simulink model "sg_2d_fir"  (Simulink 7.6)
settings: Solver=ode45  StartTime=0.0  StopTime=1600.0  RelTol=1e-3
undefined symbols (not defined in the file): gcbh, xlBlockLoadCallback, xlGetNormalizedPeriod, xlipgetpartsetting
libraries: xbsIndex_r4 x311, dspsrcs4 x6
(part 4 of 4)

== system sg_2d_fir/sg_2d_fir/5x5_Filters/Green_Filter/5x5_Filter/2D_FIR/n-tap FIR Compiler Filter4 ==
  Din : Inport
  coef : Inport  Port=2
  load : Inport  Port=3
  "FIR Compiler 5.0 " : xbsIndex_r4/FIR Compiler 5.0   coefficientvector=zeros(1,5)  coefficient_sets=1  filter_type=Single_Rate  rate_change_type=Integer  interpolation_rate=1  decimation_rate=1  zero_pack_factor=1  number_channels=1  ratespecification=Maximum_Possible  sampleperiod=1  hardwareoversamplingrate=1  filter_architecture=Systolic_Multiply_Accumulate  coefficient_reload=on  coefficient_structure=Non_Symmetric  coefficient_sign=Signed  quantization=Quantize_Only  coefficient_width=coef_n_bits  bestprecision=off  coefficient_fractional_bits=coef_bin_pt  number_paths=1  output_rounding_mode=Full_Precision  output_width=26  allow_rounding_approximation=off  optimization_goal=Area  has_sclr=off  has_data_valid=off  has_nd=off  has_ce=off  usechan_in_adv=off  chan_in_adv=0  data_buffer_type=Automatic  coefficient_buffer_type=Automatic  input_buffer_type=Automatic  output_buffer_type=Automatic  preference_for_other_storage=Automatic  multi_column_support=Disabled  columnconfig='1'  inter_column_pipe_length=4  passband_min=0.0  passband_max=0.5  stopband_min=0.5  stopband_max=1.0  filter_selection=1  gui_behaviour=Sysgen  registered_output=true  data_sign=Signed  data_width=16  data_fractional_bits=0  wrapper_available=true  ip_wrap_arbitrary_binary_point=true  ip_name=FIR Compiler  ip_version=5.0  dsptool_ready=true  ipcore_usecache=true  ipcore_useipmodelcache=true  ipcore_xco_need_fpga_part=true  port_translation_map={ 'ce' => 'en', 'sclr' => 'rst' }  run_core_at_system_period=true  ipcore_fpga_part=xlipgetpartsetting(gcb, {'virtex4', 'xc4vsx35', '-10', 'ff668'})  structural_sim=false  block_type=fir_compiler_v5_0
      settings: block_version=11.2
  Register : xbsIndex_r4/Register  init=0  rst=off  en=on  dbl_ovrd=off  block_type=register
  Register2 : xbsIndex_r4/Register  init=0  rst=off  en=off  dbl_ovrd=off  block_type=register
      settings: block_version=9.1-beta
  Rising Edge Detector1 : Subsystem
  Terminator5 : Terminator
  Out : Outport
  wires:
  "FIR Compiler 5.0 "/2 -> Terminator5/1
  Rising Edge Detector1/1(Dout) -> "FIR Compiler 5.0 "/2
  Register2/1 -> "FIR Compiler 5.0 "/3
  load/1 -> Rising Edge Detector1/1(Din), Register2/1
  Register/1 -> Out/1
  coef/1 -> "FIR Compiler 5.0 "/4
  "FIR Compiler 5.0 "/1 -> Register/1
  "FIR Compiler 5.0 "/3 -> Register/2
  Din/1 -> "FIR Compiler 5.0 "/1

== system sg_2d_fir/sg_2d_fir/5x5_Filters/Green_Filter/5x5_Filter/2D_FIR/n-tap FIR Compiler Filter5 ==
  Din : Inport
  coef : Inport  Port=2
  load : Inport  Port=3
  "FIR Compiler 5.0 " : xbsIndex_r4/FIR Compiler 5.0   coefficientvector=zeros(1,5)  coefficient_sets=1  filter_type=Single_Rate  rate_change_type=Integer  interpolation_rate=1  decimation_rate=1  zero_pack_factor=1  number_channels=1  ratespecification=Maximum_Possible  sampleperiod=1  hardwareoversamplingrate=1  filter_architecture=Systolic_Multiply_Accumulate  coefficient_reload=on  coefficient_structure=Non_Symmetric  coefficient_sign=Signed  quantization=Quantize_Only  coefficient_width=coef_n_bits  bestprecision=off  coefficient_fractional_bits=coef_bin_pt  number_paths=1  output_rounding_mode=Full_Precision  output_width=26  allow_rounding_approximation=off  optimization_goal=Area  has_sclr=off  has_data_valid=off  has_nd=off  has_ce=off  usechan_in_adv=off  chan_in_adv=0  data_buffer_type=Automatic  coefficient_buffer_type=Automatic  input_buffer_type=Automatic  output_buffer_type=Automatic  preference_for_other_storage=Automatic  multi_column_support=Disabled  columnconfig='1'  inter_column_pipe_length=4  passband_min=0.0  passband_max=0.5  stopband_min=0.5  stopband_max=1.0  filter_selection=1  gui_behaviour=Sysgen  registered_output=true  data_sign=Signed  data_width=16  data_fractional_bits=0  wrapper_available=true  ip_wrap_arbitrary_binary_point=true  ip_name=FIR Compiler  ip_version=5.0  dsptool_ready=true  ipcore_usecache=true  ipcore_useipmodelcache=true  ipcore_xco_need_fpga_part=true  port_translation_map={ 'ce' => 'en', 'sclr' => 'rst' }  run_core_at_system_period=true  ipcore_fpga_part=xlipgetpartsetting(gcb, {'virtex4', 'xc4vsx35', '-10', 'ff668'})  structural_sim=false  block_type=fir_compiler_v5_0
      settings: block_version=11.2
  Register : xbsIndex_r4/Register  init=0  rst=off  en=on  dbl_ovrd=off  block_type=register
  Register2 : xbsIndex_r4/Register  init=0  rst=off  en=off  dbl_ovrd=off  block_type=register
      settings: block_version=9.1-beta
  Rising Edge Detector1 : Subsystem
  Terminator5 : Terminator
  Out : Outport
  wires:
  Din/1 -> "FIR Compiler 5.0 "/1
  "FIR Compiler 5.0 "/3 -> Register/2
  "FIR Compiler 5.0 "/1 -> Register/1
  coef/1 -> "FIR Compiler 5.0 "/4
  Register/1 -> Out/1
  load/1 -> Register2/1, Rising Edge Detector1/1(Din)
  Register2/1 -> "FIR Compiler 5.0 "/3
  Rising Edge Detector1/1(Dout) -> "FIR Compiler 5.0 "/2
  "FIR Compiler 5.0 "/2 -> Terminator5/1

== system sg_2d_fir/sg_2d_fir/5x5_Filters/Red_Filter/5x5_Filter/2D_FIR/ABS ==
  In1 : Inport
  Mux : xbsIndex_r4/Mux  inputs=2  en=off  latency=1  precision=Full  arith_type=Unsigned  n_bits=8  bin_pt=0  quantization=Truncate  overflow=Saturate  dbl_ovrd=off  block_type=mux
      settings: xl_area=[0, 0, 0, 0, 0, 0, 0]  block_version=VER_STRING_GOES_HERE
  Negate : xbsIndex_r4/Negate  precision=Full  arith_type=Unsigned  n_bits=8  bin_pt=2  quantization=Truncate  overflow=Wrap  en=off  latency=1  dbl_ovrd=off  block_type=negate
      settings: xl_area=[0, 0, 0, 0, 0, 0, 0]  block_version=VER_STRING_GOES_HERE
  Register1 : xbsIndex_r4/Register  init=0  rst=off  en=off  dbl_ovrd=off  block_type=register
      settings: xl_area=[0, 0, 0, 0, 0, 0, 0]  block_version=VER_STRING_GOES_HERE
  Register2 : xbsIndex_r4/Register  init=0  rst=off  en=off  dbl_ovrd=off  block_type=register
      settings: xl_area=[0, 0, 0, 0, 0, 0, 0]  block_version=VER_STRING_GOES_HERE
  Slice : xbsIndex_r4/Slice  nbits=1  boolean_output=off  mode=Upper Bit Location + Width  bit1=0  base1=MSB of Input  bit0=0  base0=LSB of Input  dbl_ovrd=off  block_type=slice
      settings: infoedit="Extracts a given range of bits from each input sample and presents it at the output.  The output type is ordinarily unsigned with binary point at zero, but can be Boolean when the slice is one bit wide.<P><P>Hardware notes: In hardware this block costs nothing."  block_version=VER_STRING_GOES_HERE
  Out1 : Outport
  wires:
  Register1/1 -> Mux/2
  Register2/1 -> Mux/1
  Mux/1 -> Out1/1
  In1/1 -> Register1/1, Slice/1, Negate/1
  Negate/1 -> Mux/3
  Slice/1 -> Register2/1

== system sg_2d_fir/sg_2d_fir/5x5_Filters/Red_Filter/5x5_Filter/2D_FIR/n-tap FIR Compiler Filter1 ==
  Din : Inport
  coef : Inport  Port=2
  load : Inport  Port=3
  "FIR Compiler 5.0 " : xbsIndex_r4/FIR Compiler 5.0   coefficientvector=zeros(1,5)  coefficient_sets=1  filter_type=Single_Rate  rate_change_type=Integer  interpolation_rate=1  decimation_rate=1  zero_pack_factor=1  number_channels=1  ratespecification=Maximum_Possible  sampleperiod=1  hardwareoversamplingrate=1  filter_architecture=Systolic_Multiply_Accumulate  coefficient_reload=on  coefficient_structure=Non_Symmetric  coefficient_sign=Signed  quantization=Quantize_Only  coefficient_width=coef_n_bits  bestprecision=off  coefficient_fractional_bits=coef_bin_pt  number_paths=1  output_rounding_mode=Full_Precision  output_width=26  allow_rounding_approximation=off  optimization_goal=Area  has_sclr=off  has_data_valid=off  has_nd=off  has_ce=off  usechan_in_adv=off  chan_in_adv=0  data_buffer_type=Automatic  coefficient_buffer_type=Automatic  input_buffer_type=Automatic  output_buffer_type=Automatic  preference_for_other_storage=Automatic  multi_column_support=Disabled  columnconfig='1'  inter_column_pipe_length=4  passband_min=0.0  passband_max=0.5  stopband_min=0.5  stopband_max=1.0  filter_selection=1  gui_behaviour=Sysgen  registered_output=true  data_sign=Signed  data_width=16  data_fractional_bits=0  wrapper_available=true  ip_wrap_arbitrary_binary_point=true  ip_name=FIR Compiler  ip_version=5.0  dsptool_ready=true  ipcore_usecache=true  ipcore_useipmodelcache=true  ipcore_xco_need_fpga_part=true  port_translation_map={ 'ce' => 'en', 'sclr' => 'rst' }  run_core_at_system_period=true  ipcore_fpga_part=xlipgetpartsetting(gcb, {'virtex4', 'xc4vsx35', '-10', 'ff668'})  structural_sim=false  block_type=fir_compiler_v5_0
      settings: block_version=11.2
  Register : xbsIndex_r4/Register  init=0  rst=off  en=on  dbl_ovrd=off  block_type=register
  Register2 : xbsIndex_r4/Register  init=0  rst=off  en=off  dbl_ovrd=off  block_type=register
      settings: block_version=9.1-beta
  Rising Edge Detector1 : Subsystem
  Terminator5 : Terminator
  Out : Outport
  wires:
  "FIR Compiler 5.0 "/2 -> Terminator5/1
  Rising Edge Detector1/1(Dout) -> "FIR Compiler 5.0 "/2
  Register2/1 -> "FIR Compiler 5.0 "/3
  load/1 -> Rising Edge Detector1/1(Din), Register2/1
  Register/1 -> Out/1
  coef/1 -> "FIR Compiler 5.0 "/4
  "FIR Compiler 5.0 "/1 -> Register/1
  "FIR Compiler 5.0 "/3 -> Register/2
  Din/1 -> "FIR Compiler 5.0 "/1

== system sg_2d_fir/sg_2d_fir/5x5_Filters/Red_Filter/5x5_Filter/2D_FIR/n-tap FIR Compiler Filter2 ==
  Din : Inport
  coef : Inport  Port=2
  load : Inport  Port=3
  "FIR Compiler 5.0 " : xbsIndex_r4/FIR Compiler 5.0   coefficientvector=zeros(1,5)  coefficient_sets=1  filter_type=Single_Rate  rate_change_type=Integer  interpolation_rate=1  decimation_rate=1  zero_pack_factor=1  number_channels=1  ratespecification=Maximum_Possible  sampleperiod=1  hardwareoversamplingrate=1  filter_architecture=Systolic_Multiply_Accumulate  coefficient_reload=on  coefficient_structure=Non_Symmetric  coefficient_sign=Signed  quantization=Quantize_Only  coefficient_width=coef_n_bits  bestprecision=off  coefficient_fractional_bits=coef_bin_pt  number_paths=1  output_rounding_mode=Full_Precision  output_width=26  allow_rounding_approximation=off  optimization_goal=Area  has_sclr=off  has_data_valid=off  has_nd=off  has_ce=off  usechan_in_adv=off  chan_in_adv=0  data_buffer_type=Automatic  coefficient_buffer_type=Automatic  input_buffer_type=Automatic  output_buffer_type=Automatic  preference_for_other_storage=Automatic  multi_column_support=Disabled  columnconfig='1'  inter_column_pipe_length=4  passband_min=0.0  passband_max=0.5  stopband_min=0.5  stopband_max=1.0  filter_selection=1  gui_behaviour=Sysgen  registered_output=true  data_sign=Signed  data_width=16  data_fractional_bits=0  wrapper_available=true  ip_wrap_arbitrary_binary_point=true  ip_name=FIR Compiler  ip_version=5.0  dsptool_ready=true  ipcore_usecache=true  ipcore_useipmodelcache=true  ipcore_xco_need_fpga_part=true  port_translation_map={ 'ce' => 'en', 'sclr' => 'rst' }  run_core_at_system_period=true  ipcore_fpga_part=xlipgetpartsetting(gcb, {'virtex4', 'xc4vsx35', '-10', 'ff668'})  structural_sim=false  block_type=fir_compiler_v5_0
      settings: block_version=11.2
  Register : xbsIndex_r4/Register  init=0  rst=off  en=on  dbl_ovrd=off  block_type=register
  Register2 : xbsIndex_r4/Register  init=0  rst=off  en=off  dbl_ovrd=off  block_type=register
      settings: block_version=9.1-beta
  Rising Edge Detector1 : Subsystem
  Terminator5 : Terminator
  Out : Outport
  wires:
  Din/1 -> "FIR Compiler 5.0 "/1
  "FIR Compiler 5.0 "/3 -> Register/2
  "FIR Compiler 5.0 "/1 -> Register/1
  coef/1 -> "FIR Compiler 5.0 "/4
  Register/1 -> Out/1
  load/1 -> Register2/1, Rising Edge Detector1/1(Din)
  Register2/1 -> "FIR Compiler 5.0 "/3
  Rising Edge Detector1/1(Dout) -> "FIR Compiler 5.0 "/2
  "FIR Compiler 5.0 "/2 -> Terminator5/1

== system sg_2d_fir/sg_2d_fir/5x5_Filters/Red_Filter/5x5_Filter/2D_FIR/n-tap FIR Compiler Filter3 ==
  Din : Inport
  coef : Inport  Port=2
  load : Inport  Port=3
  "FIR Compiler 5.0 " : xbsIndex_r4/FIR Compiler 5.0   coefficientvector=zeros(1,5)  coefficient_sets=1  filter_type=Single_Rate  rate_change_type=Integer  interpolation_rate=1  decimation_rate=1  zero_pack_factor=1  number_channels=1  ratespecification=Maximum_Possible  sampleperiod=1  hardwareoversamplingrate=1  filter_architecture=Systolic_Multiply_Accumulate  coefficient_reload=on  coefficient_structure=Non_Symmetric  coefficient_sign=Signed  quantization=Quantize_Only  coefficient_width=coef_n_bits  bestprecision=off  coefficient_fractional_bits=coef_bin_pt  number_paths=1  output_rounding_mode=Full_Precision  output_width=26  allow_rounding_approximation=off  optimization_goal=Area  has_sclr=off  has_data_valid=off  has_nd=off  has_ce=off  usechan_in_adv=off  chan_in_adv=0  data_buffer_type=Automatic  coefficient_buffer_type=Automatic  input_buffer_type=Automatic  output_buffer_type=Automatic  preference_for_other_storage=Automatic  multi_column_support=Disabled  columnconfig='1'  inter_column_pipe_length=4  passband_min=0.0  passband_max=0.5  stopband_min=0.5  stopband_max=1.0  filter_selection=1  gui_behaviour=Sysgen  registered_output=true  data_sign=Signed  data_width=16  data_fractional_bits=0  wrapper_available=true  ip_wrap_arbitrary_binary_point=true  ip_name=FIR Compiler  ip_version=5.0  dsptool_ready=true  ipcore_usecache=true  ipcore_useipmodelcache=true  ipcore_xco_need_fpga_part=true  port_translation_map={ 'ce' => 'en', 'sclr' => 'rst' }  run_core_at_system_period=true  ipcore_fpga_part=xlipgetpartsetting(gcb, {'virtex4', 'xc4vsx35', '-10', 'ff668'})  structural_sim=false  block_type=fir_compiler_v5_0
      settings: block_version=11.2
  Register : xbsIndex_r4/Register  init=0  rst=off  en=on  dbl_ovrd=off  block_type=register
  Register2 : xbsIndex_r4/Register  init=0  rst=off  en=off  dbl_ovrd=off  block_type=register
      settings: block_version=9.1-beta
  Rising Edge Detector1 : Subsystem
  Terminator5 : Terminator
  Out : Outport
  wires:
  "FIR Compiler 5.0 "/2 -> Terminator5/1
  Rising Edge Detector1/1(Dout) -> "FIR Compiler 5.0 "/2
  Register2/1 -> "FIR Compiler 5.0 "/3
  load/1 -> Rising Edge Detector1/1(Din), Register2/1
  Register/1 -> Out/1
  coef/1 -> "FIR Compiler 5.0 "/4
  "FIR Compiler 5.0 "/1 -> Register/1
  "FIR Compiler 5.0 "/3 -> Register/2
  Din/1 -> "FIR Compiler 5.0 "/1

== system sg_2d_fir/sg_2d_fir/5x5_Filters/Red_Filter/5x5_Filter/2D_FIR/n-tap FIR Compiler Filter4 ==
  Din : Inport
  coef : Inport  Port=2
  load : Inport  Port=3
  "FIR Compiler 5.0 " : xbsIndex_r4/FIR Compiler 5.0   coefficientvector=zeros(1,5)  coefficient_sets=1  filter_type=Single_Rate  rate_change_type=Integer  interpolation_rate=1  decimation_rate=1  zero_pack_factor=1  number_channels=1  ratespecification=Maximum_Possible  sampleperiod=1  hardwareoversamplingrate=1  filter_architecture=Systolic_Multiply_Accumulate  coefficient_reload=on  coefficient_structure=Non_Symmetric  coefficient_sign=Signed  quantization=Quantize_Only  coefficient_width=coef_n_bits  bestprecision=off  coefficient_fractional_bits=coef_bin_pt  number_paths=1  output_rounding_mode=Full_Precision  output_width=26  allow_rounding_approximation=off  optimization_goal=Area  has_sclr=off  has_data_valid=off  has_nd=off  has_ce=off  usechan_in_adv=off  chan_in_adv=0  data_buffer_type=Automatic  coefficient_buffer_type=Automatic  input_buffer_type=Automatic  output_buffer_type=Automatic  preference_for_other_storage=Automatic  multi_column_support=Disabled  columnconfig='1'  inter_column_pipe_length=4  passband_min=0.0  passband_max=0.5  stopband_min=0.5  stopband_max=1.0  filter_selection=1  gui_behaviour=Sysgen  registered_output=true  data_sign=Signed  data_width=16  data_fractional_bits=0  wrapper_available=true  ip_wrap_arbitrary_binary_point=true  ip_name=FIR Compiler  ip_version=5.0  dsptool_ready=true  ipcore_usecache=true  ipcore_useipmodelcache=true  ipcore_xco_need_fpga_part=true  port_translation_map={ 'ce' => 'en', 'sclr' => 'rst' }  run_core_at_system_period=true  ipcore_fpga_part=xlipgetpartsetting(gcb, {'virtex4', 'xc4vsx35', '-10', 'ff668'})  structural_sim=false  block_type=fir_compiler_v5_0
      settings: block_version=11.2
  Register : xbsIndex_r4/Register  init=0  rst=off  en=on  dbl_ovrd=off  block_type=register
  Register2 : xbsIndex_r4/Register  init=0  rst=off  en=off  dbl_ovrd=off  block_type=register
      settings: block_version=9.1-beta
  Rising Edge Detector1 : Subsystem
  Terminator5 : Terminator
  Out : Outport
  wires:
  Din/1 -> "FIR Compiler 5.0 "/1
  "FIR Compiler 5.0 "/3 -> Register/2
  "FIR Compiler 5.0 "/1 -> Register/1
  coef/1 -> "FIR Compiler 5.0 "/4
  Register/1 -> Out/1
  load/1 -> Register2/1, Rising Edge Detector1/1(Din)
  Register2/1 -> "FIR Compiler 5.0 "/3
  Rising Edge Detector1/1(Dout) -> "FIR Compiler 5.0 "/2
  "FIR Compiler 5.0 "/2 -> Terminator5/1

== system sg_2d_fir/sg_2d_fir/5x5_Filters/Red_Filter/5x5_Filter/2D_FIR/n-tap FIR Compiler Filter5 ==
  Din : Inport
  coef : Inport  Port=2
  load : Inport  Port=3
  "FIR Compiler 5.0 " : xbsIndex_r4/FIR Compiler 5.0   coefficientvector=zeros(1,5)  coefficient_sets=1  filter_type=Single_Rate  rate_change_type=Integer  interpolation_rate=1  decimation_rate=1  zero_pack_factor=1  number_channels=1  ratespecification=Maximum_Possible  sampleperiod=1  hardwareoversamplingrate=1  filter_architecture=Systolic_Multiply_Accumulate  coefficient_reload=on  coefficient_structure=Non_Symmetric  coefficient_sign=Signed  quantization=Quantize_Only  coefficient_width=coef_n_bits  bestprecision=off  coefficient_fractional_bits=coef_bin_pt  number_paths=1  output_rounding_mode=Full_Precision  output_width=26  allow_rounding_approximation=off  optimization_goal=Area  has_sclr=off  has_data_valid=off  has_nd=off  has_ce=off  usechan_in_adv=off  chan_in_adv=0  data_buffer_type=Automatic  coefficient_buffer_type=Automatic  input_buffer_type=Automatic  output_buffer_type=Automatic  preference_for_other_storage=Automatic  multi_column_support=Disabled  columnconfig='1'  inter_column_pipe_length=4  passband_min=0.0  passband_max=0.5  stopband_min=0.5  stopband_max=1.0  filter_selection=1  gui_behaviour=Sysgen  registered_output=true  data_sign=Signed  data_width=16  data_fractional_bits=0  wrapper_available=true  ip_wrap_arbitrary_binary_point=true  ip_name=FIR Compiler  ip_version=5.0  dsptool_ready=true  ipcore_usecache=true  ipcore_useipmodelcache=true  ipcore_xco_need_fpga_part=true  port_translation_map={ 'ce' => 'en', 'sclr' => 'rst' }  run_core_at_system_period=true  ipcore_fpga_part=xlipgetpartsetting(gcb, {'virtex4', 'xc4vsx35', '-10', 'ff668'})  structural_sim=false  block_type=fir_compiler_v5_0
      settings: block_version=11.2
  Register : xbsIndex_r4/Register  init=0  rst=off  en=on  dbl_ovrd=off  block_type=register
  Register2 : xbsIndex_r4/Register  init=0  rst=off  en=off  dbl_ovrd=off  block_type=register
      settings: block_version=9.1-beta
  Rising Edge Detector1 : Subsystem
  Terminator5 : Terminator
  Out : Outport
  wires:
  "FIR Compiler 5.0 "/2 -> Terminator5/1
  Rising Edge Detector1/1(Dout) -> "FIR Compiler 5.0 "/2
  Register2/1 -> "FIR Compiler 5.0 "/3
  load/1 -> Rising Edge Detector1/1(Din), Register2/1
  Register/1 -> Out/1
  coef/1 -> "FIR Compiler 5.0 "/4
  "FIR Compiler 5.0 "/1 -> Register/1
  "FIR Compiler 5.0 "/3 -> Register/2
  Din/1 -> "FIR Compiler 5.0 "/1

== system sg_2d_fir/sg_2d_fir/5x5_Filters/Blue_Filter/5x5_Filter/2D_FIR/n-tap FIR Compiler Filter1/Rising Edge Detector1 ==
  Din : Inport
  Inverter : xbsIndex_r4/Inverter  en=off  latency=0  dbl_ovrd=off  block_type=inv
      settings: block_version=9.1
  Logical : xbsIndex_r4/Logical  logical_function=AND  inputs=2  en=off  latency=0  precision=Full  arith_type=Unsigned  n_bits=16  bin_pt=0  align_bp=on  dbl_ovrd=off  block_type=logical
      settings: block_version=9.1
  Register1 : xbsIndex_r4/Register  init=0  rst=off  en=off  dbl_ovrd=off  block_type=register
      settings: block_version=9.1
  Dout : Outport
  wires:
  Logical/1 -> Dout/1
  Din/1 -> Register1/1, Logical/1
  Inverter/1 -> Logical/2
  Register1/1 -> Inverter/1

== system sg_2d_fir/sg_2d_fir/5x5_Filters/Blue_Filter/5x5_Filter/2D_FIR/n-tap FIR Compiler Filter2/Rising Edge Detector1 ==
  Din : Inport
  Inverter : xbsIndex_r4/Inverter  en=off  latency=0  dbl_ovrd=off  block_type=inv
      settings: block_version=9.1
  Logical : xbsIndex_r4/Logical  logical_function=AND  inputs=2  en=off  latency=0  precision=Full  arith_type=Unsigned  n_bits=16  bin_pt=0  align_bp=on  dbl_ovrd=off  block_type=logical
      settings: block_version=9.1
  Register1 : xbsIndex_r4/Register  init=0  rst=off  en=off  dbl_ovrd=off  block_type=register
      settings: block_version=9.1
  Dout : Outport
  wires:
  Register1/1 -> Inverter/1
  Inverter/1 -> Logical/2
  Din/1 -> Logical/1, Register1/1
  Logical/1 -> Dout/1

== system sg_2d_fir/sg_2d_fir/5x5_Filters/Blue_Filter/5x5_Filter/2D_FIR/n-tap FIR Compiler Filter3/Rising Edge Detector1 ==
  Din : Inport
  Inverter : xbsIndex_r4/Inverter  en=off  latency=0  dbl_ovrd=off  block_type=inv
      settings: block_version=9.1
  Logical : xbsIndex_r4/Logical  logical_function=AND  inputs=2  en=off  latency=0  precision=Full  arith_type=Unsigned  n_bits=16  bin_pt=0  align_bp=on  dbl_ovrd=off  block_type=logical
      settings: block_version=9.1
  Register1 : xbsIndex_r4/Register  init=0  rst=off  en=off  dbl_ovrd=off  block_type=register
      settings: block_version=9.1
  Dout : Outport
  wires:
  Logical/1 -> Dout/1
  Din/1 -> Register1/1, Logical/1
  Inverter/1 -> Logical/2
  Register1/1 -> Inverter/1

== system sg_2d_fir/sg_2d_fir/5x5_Filters/Blue_Filter/5x5_Filter/2D_FIR/n-tap FIR Compiler Filter4/Rising Edge Detector1 ==
  Din : Inport
  Inverter : xbsIndex_r4/Inverter  en=off  latency=0  dbl_ovrd=off  block_type=inv
      settings: block_version=9.1
  Logical : xbsIndex_r4/Logical  logical_function=AND  inputs=2  en=off  latency=0  precision=Full  arith_type=Unsigned  n_bits=16  bin_pt=0  align_bp=on  dbl_ovrd=off  block_type=logical
      settings: block_version=9.1
  Register1 : xbsIndex_r4/Register  init=0  rst=off  en=off  dbl_ovrd=off  block_type=register
      settings: block_version=9.1
  Dout : Outport
  wires:
  Register1/1 -> Inverter/1
  Inverter/1 -> Logical/2
  Din/1 -> Logical/1, Register1/1
  Logical/1 -> Dout/1

== system sg_2d_fir/sg_2d_fir/5x5_Filters/Blue_Filter/5x5_Filter/2D_FIR/n-tap FIR Compiler Filter5/Rising Edge Detector1 ==
  Din : Inport
  Inverter : xbsIndex_r4/Inverter  en=off  latency=0  dbl_ovrd=off  block_type=inv
      settings: block_version=9.1
  Logical : xbsIndex_r4/Logical  logical_function=AND  inputs=2  en=off  latency=0  precision=Full  arith_type=Unsigned  n_bits=16  bin_pt=0  align_bp=on  dbl_ovrd=off  block_type=logical
      settings: block_version=9.1
  Register1 : xbsIndex_r4/Register  init=0  rst=off  en=off  dbl_ovrd=off  block_type=register
      settings: block_version=9.1
  Dout : Outport
  wires:
  Logical/1 -> Dout/1
  Din/1 -> Register1/1, Logical/1
  Inverter/1 -> Logical/2
  Register1/1 -> Inverter/1

== system sg_2d_fir/sg_2d_fir/5x5_Filters/Green_Filter/5x5_Filter/2D_FIR/n-tap FIR Compiler Filter1/Rising Edge Detector1 ==
  Din : Inport
  Inverter : xbsIndex_r4/Inverter  en=off  latency=0  dbl_ovrd=off  block_type=inv
      settings: block_version=9.1
  Logical : xbsIndex_r4/Logical  logical_function=AND  inputs=2  en=off  latency=0  precision=Full  arith_type=Unsigned  n_bits=16  bin_pt=0  align_bp=on  dbl_ovrd=off  block_type=logical
      settings: block_version=9.1
  Register1 : xbsIndex_r4/Register  init=0  rst=off  en=off  dbl_ovrd=off  block_type=register
      settings: block_version=9.1
  Dout : Outport
  wires:
  Logical/1 -> Dout/1
  Din/1 -> Register1/1, Logical/1
  Inverter/1 -> Logical/2
  Register1/1 -> Inverter/1

== system sg_2d_fir/sg_2d_fir/5x5_Filters/Green_Filter/5x5_Filter/2D_FIR/n-tap FIR Compiler Filter2/Rising Edge Detector1 ==
  Din : Inport
  Inverter : xbsIndex_r4/Inverter  en=off  latency=0  dbl_ovrd=off  block_type=inv
      settings: block_version=9.1
  Logical : xbsIndex_r4/Logical  logical_function=AND  inputs=2  en=off  latency=0  precision=Full  arith_type=Unsigned  n_bits=16  bin_pt=0  align_bp=on  dbl_ovrd=off  block_type=logical
      settings: block_version=9.1
  Register1 : xbsIndex_r4/Register  init=0  rst=off  en=off  dbl_ovrd=off  block_type=register
      settings: block_version=9.1
  Dout : Outport
  wires:
  Register1/1 -> Inverter/1
  Inverter/1 -> Logical/2
  Din/1 -> Logical/1, Register1/1
  Logical/1 -> Dout/1

== system sg_2d_fir/sg_2d_fir/5x5_Filters/Green_Filter/5x5_Filter/2D_FIR/n-tap FIR Compiler Filter3/Rising Edge Detector1 ==
  Din : Inport
  Inverter : xbsIndex_r4/Inverter  en=off  latency=0  dbl_ovrd=off  block_type=inv
      settings: block_version=9.1
  Logical : xbsIndex_r4/Logical  logical_function=AND  inputs=2  en=off  latency=0  precision=Full  arith_type=Unsigned  n_bits=16  bin_pt=0  align_bp=on  dbl_ovrd=off  block_type=logical
      settings: block_version=9.1
  Register1 : xbsIndex_r4/Register  init=0  rst=off  en=off  dbl_ovrd=off  block_type=register
      settings: block_version=9.1
  Dout : Outport
  wires:
  Logical/1 -> Dout/1
  Din/1 -> Register1/1, Logical/1
  Inverter/1 -> Logical/2
  Register1/1 -> Inverter/1

== system sg_2d_fir/sg_2d_fir/5x5_Filters/Green_Filter/5x5_Filter/2D_FIR/n-tap FIR Compiler Filter4/Rising Edge Detector1 ==
  Din : Inport
  Inverter : xbsIndex_r4/Inverter  en=off  latency=0  dbl_ovrd=off  block_type=inv
      settings: block_version=9.1
  Logical : xbsIndex_r4/Logical  logical_function=AND  inputs=2  en=off  latency=0  precision=Full  arith_type=Unsigned  n_bits=16  bin_pt=0  align_bp=on  dbl_ovrd=off  block_type=logical
      settings: block_version=9.1
  Register1 : xbsIndex_r4/Register  init=0  rst=off  en=off  dbl_ovrd=off  block_type=register
      settings: block_version=9.1
  Dout : Outport
  wires:
  Register1/1 -> Inverter/1
  Inverter/1 -> Logical/2
  Din/1 -> Logical/1, Register1/1
  Logical/1 -> Dout/1

== system sg_2d_fir/sg_2d_fir/5x5_Filters/Green_Filter/5x5_Filter/2D_FIR/n-tap FIR Compiler Filter5/Rising Edge Detector1 ==
  Din : Inport
  Inverter : xbsIndex_r4/Inverter  en=off  latency=0  dbl_ovrd=off  block_type=inv
      settings: block_version=9.1
  Logical : xbsIndex_r4/Logical  logical_function=AND  inputs=2  en=off  latency=0  precision=Full  arith_type=Unsigned  n_bits=16  bin_pt=0  align_bp=on  dbl_ovrd=off  block_type=logical
      settings: block_version=9.1
  Register1 : xbsIndex_r4/Register  init=0  rst=off  en=off  dbl_ovrd=off  block_type=register
      settings: block_version=9.1
  Dout : Outport
  wires:
  Logical/1 -> Dout/1
  Din/1 -> Register1/1, Logical/1
  Inverter/1 -> Logical/2
  Register1/1 -> Inverter/1

== system sg_2d_fir/sg_2d_fir/5x5_Filters/Red_Filter/5x5_Filter/2D_FIR/n-tap FIR Compiler Filter1/Rising Edge Detector1 ==
  Din : Inport
  Inverter : xbsIndex_r4/Inverter  en=off  latency=0  dbl_ovrd=off  block_type=inv
      settings: block_version=9.1
  Logical : xbsIndex_r4/Logical  logical_function=AND  inputs=2  en=off  latency=0  precision=Full  arith_type=Unsigned  n_bits=16  bin_pt=0  align_bp=on  dbl_ovrd=off  block_type=logical
      settings: block_version=9.1
  Register1 : xbsIndex_r4/Register  init=0  rst=off  en=off  dbl_ovrd=off  block_type=register
      settings: block_version=9.1
  Dout : Outport
  wires:
  Register1/1 -> Inverter/1
  Inverter/1 -> Logical/2
  Din/1 -> Logical/1, Register1/1
  Logical/1 -> Dout/1

== system sg_2d_fir/sg_2d_fir/5x5_Filters/Red_Filter/5x5_Filter/2D_FIR/n-tap FIR Compiler Filter2/Rising Edge Detector1 ==
  Din : Inport
  Inverter : xbsIndex_r4/Inverter  en=off  latency=0  dbl_ovrd=off  block_type=inv
      settings: block_version=9.1
  Logical : xbsIndex_r4/Logical  logical_function=AND  inputs=2  en=off  latency=0  precision=Full  arith_type=Unsigned  n_bits=16  bin_pt=0  align_bp=on  dbl_ovrd=off  block_type=logical
      settings: block_version=9.1
  Register1 : xbsIndex_r4/Register  init=0  rst=off  en=off  dbl_ovrd=off  block_type=register
      settings: block_version=9.1
  Dout : Outport
  wires:
  Logical/1 -> Dout/1
  Din/1 -> Register1/1, Logical/1
  Inverter/1 -> Logical/2
  Register1/1 -> Inverter/1

== system sg_2d_fir/sg_2d_fir/5x5_Filters/Red_Filter/5x5_Filter/2D_FIR/n-tap FIR Compiler Filter3/Rising Edge Detector1 ==
  Din : Inport
  Inverter : xbsIndex_r4/Inverter  en=off  latency=0  dbl_ovrd=off  block_type=inv
      settings: block_version=9.1
  Logical : xbsIndex_r4/Logical  logical_function=AND  inputs=2  en=off  latency=0  precision=Full  arith_type=Unsigned  n_bits=16  bin_pt=0  align_bp=on  dbl_ovrd=off  block_type=logical
      settings: block_version=9.1
  Register1 : xbsIndex_r4/Register  init=0  rst=off  en=off  dbl_ovrd=off  block_type=register
      settings: block_version=9.1
  Dout : Outport
  wires:
  Register1/1 -> Inverter/1
  Inverter/1 -> Logical/2
  Din/1 -> Logical/1, Register1/1
  Logical/1 -> Dout/1

== system sg_2d_fir/sg_2d_fir/5x5_Filters/Red_Filter/5x5_Filter/2D_FIR/n-tap FIR Compiler Filter4/Rising Edge Detector1 ==
  Din : Inport
  Inverter : xbsIndex_r4/Inverter  en=off  latency=0  dbl_ovrd=off  block_type=inv
      settings: block_version=9.1
  Logical : xbsIndex_r4/Logical  logical_function=AND  inputs=2  en=off  latency=0  precision=Full  arith_type=Unsigned  n_bits=16  bin_pt=0  align_bp=on  dbl_ovrd=off  block_type=logical
      settings: block_version=9.1
  Register1 : xbsIndex_r4/Register  init=0  rst=off  en=off  dbl_ovrd=off  block_type=register
      settings: block_version=9.1
  Dout : Outport
  wires:
  Logical/1 -> Dout/1
  Din/1 -> Register1/1, Logical/1
  Inverter/1 -> Logical/2
  Register1/1 -> Inverter/1

== system sg_2d_fir/sg_2d_fir/5x5_Filters/Red_Filter/5x5_Filter/2D_FIR/n-tap FIR Compiler Filter5/Rising Edge Detector1 ==
  Din : Inport
  Inverter : xbsIndex_r4/Inverter  en=off  latency=0  dbl_ovrd=off  block_type=inv
      settings: block_version=9.1
  Logical : xbsIndex_r4/Logical  logical_function=AND  inputs=2  en=off  latency=0  precision=Full  arith_type=Unsigned  n_bits=16  bin_pt=0  align_bp=on  dbl_ovrd=off  block_type=logical
      settings: block_version=9.1
  Register1 : xbsIndex_r4/Register  init=0  rst=off  en=off  dbl_ovrd=off  block_type=register
      settings: block_version=9.1
  Dout : Outport
  wires:
  Register1/1 -> Inverter/1
  Inverter/1 -> Logical/2
  Din/1 -> Logical/1, Register1/1
  Logical/1 -> Dout/1
